simulink model "symulacjaPID"  (R2017b)
settings: Solver=VariableStepAuto  StartTime=0.0  StopTime=10.0  RelTol=1e-3
values from neighbouring files (symbols this model uses):
  Asy = 1    [projekt2.m]
  Asy2 = 1    [projekt2.m]
  Asz = -0.1    [projekt2.m]
  Ay = 1    [projekt2.m]
  Ay2 = 1    [projekt2.m]
  Az = 0.1    [projekt2.m]
  fazay = pi/2    (= 1.57079632679)    [projekt2.m]
  fazay2 = 0    [projekt2.m]
  fazaz = 0    [projekt2.m]
  K = 1.4    [projekt2.m]
  kd = 6    [projekt2.m]
  Kp = 0.3894    [projekt2.m]
  omy = 0.05    [projekt2.m]
  omy2 = 0.01    [projekt2.m]
  omz = 0.05    [projekt2.m]
  T1 = 1/14    (= 0.0714285714286)    [projekt2.m]
  T2 = 100    [projekt2.m]
  T3 = 10    [projekt2.m]
  T4 = 1    [projekt2.m]
  Td = 9    [projekt2.m]
  Ti = 36    [projekt2.m]
  Ty = 10    [projekt2.m]
  Ty2 = 10    [projekt2.m]
  Tz = 0    [projekt2.m]
settings Model: Creator=Alicja  LastModifiedBy=Alicja
settings DataIOCC: SaveFormat=Array  OutputSaveName=z, y, yr, ur, e

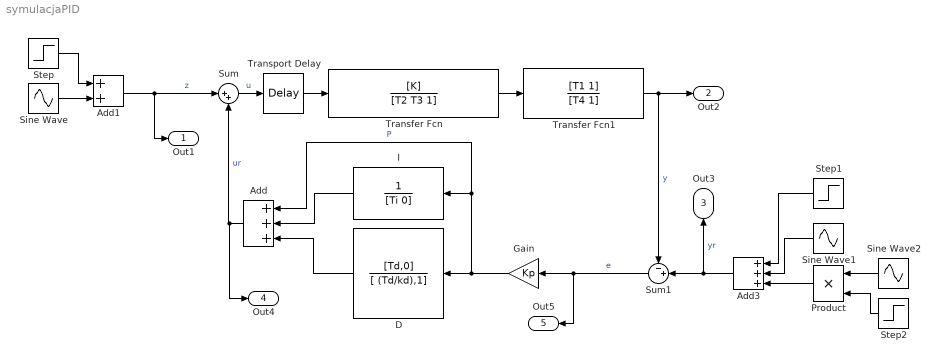
== system symulacjaPID ==
  Add : Sum  Inputs=+++
  Add1 : Sum  OutDataTypeStr=Inherit: Same as first input
  Add3 : Sum  Inputs=+++  OutDataTypeStr=Inherit: Same as first input
  D : TransferFcn  Numerator=[Td,0]  Denominator=[ (Td/kd),1]
  Gain : Gain  Gain=Kp
  I : TransferFcn  Denominator=[Ti 0]
  Product : Product
  Sine Wave : Sin  Amplitude=Asz  Frequency=omz  Phase=fazaz  SampleTime=0
  Sine Wave1 : Sin  Amplitude=Asy  Frequency=omy  Phase=fazay  SampleTime=0
  Sine Wave2 : Sin  Amplitude=Asy2  Frequency=omy2  Phase=fazay2  SampleTime=0
  Step : Step  Time=Tz  After=Az  SampleTime=0
  Step1 : Step  Time=Ty  After=Ay  SampleTime=0
  Step2 : Step  Time=Ty2  After=Ay2  SampleTime=0
  Sum : Sum  Inputs=|++
  Sum1 : Sum  Inputs=-+|
  Transfer Fcn : TransferFcn  Numerator=[K]  Denominator=[T2 T3 1]
  Transfer Fcn1 : TransferFcn  Numerator=[T1 1]  Denominator=[T4 1]
  Transport Delay : TransportDelay  DelayTime=20
  Out1 : Outport
  Out2 : Outport  Port=2
  Out3 : Outport  Port=3
  Out4 : Outport  Port=4
  Out5 : Outport  Port=5
  wires:
  Sum1/1 -> Out5/1, Gain/1  "e"
  Sum/1 -> Transport Delay/1  "u"
  Add/1 -> Out4/1, Sum/2  "ur"
  Add1/1 -> Out1/1, Sum/1  "z"
  Transfer Fcn1/1 -> Out2/1, Sum1/1  "y"
  Transport Delay/1 -> Transfer Fcn/1
  I/1 -> Add/2
  D/1 -> Add/3
  Gain/1 -> D/1, I/1, Add/1  "P"
  Add3/1 -> Sum1/2, Out3/1  "yr"
  Sine Wave/1 -> Add1/2
  Step/1 -> Add1/1
  Step1/1 -> Add3/1
  Sine Wave1/1 -> Add3/2
  Transfer Fcn/1 -> Transfer Fcn1/1
  Sine Wave2/1 -> Product/1
  Step2/1 -> Product/2
  Product/1 -> Add3/3
